simulink model "pendule_simple"  (R2023a)
settings: Solver=VariableStepAuto  StartTime=0.0  StopTime=10.0  RelTol=1e-3
undefined symbols (not defined in the file): g, l
settings Model: Creator=crt4254  LastModifiedBy=crt4254

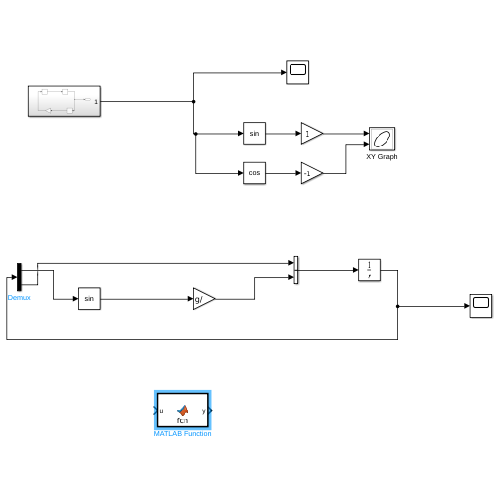
[thumbnail: Simulink's stored preview of the top-level diagram]
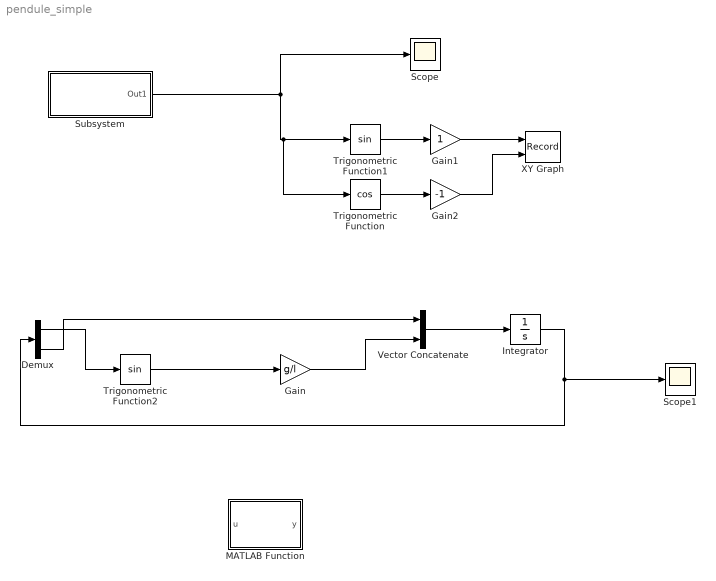
== system pendule_simple ==
  Demux : Demux  Outputs=2
  Gain : Gain  Gain=g/l
  Gain1 : Gain
  Gain2 : Gain  Gain=-1
  Integrator : Integrator  InitialCondition=[1 pi]
  MATLAB Function : MATLAB Function  TreatAsAtomicUnit=on
  Scope : Scope
  Scope1 : Scope
  Subsystem : Subsystem
  Trigonometric Function : Trigonometry  Operator=cos
  Trigonometric Function1 : Trigonometry
  Trigonometric Function2 : Trigonometry
  Vector Concatenate : Concatenate
  XY Graph : Record  FileSettingsInternal="{\"entries\":[{\"content\":{\"excelSettings\":{\"content\":{},\"type\":\"Streamout.ExcelSettings\"}},\"type\":\"Streamout.FileSettingStorage\",\"uuid\":\"855e007d-fd6a-4001-b943-7c5d9cd4a3f9\"}],\"packageUris\":[\"http://schema.mathworks.com/mf0/streamout_blocks/R2020a\"],\"version\":\"1.0\"}"  Layout=[1 1]  SignalsInternal="{\"entries\":[{\"content\":{\"signals\":[{\"content\":{\"blockPath\":[\"pendule_simple/XY Graph\"],\"dimensions\":[1],\"domain\":\"pendule_simple/XY Graph\",\"lineColor\":\"#a2142f\",\"plots\":[1],\"port\":1,\"sid\":[\"\"],\"signalID\":149,\"signalName\":\"Gain1\"},\"type\":\"RecordBlkView.Signal\",\"uuid\":\"53e22b2f-952e-4340-82ff-a1eee0395188\"},{\"content\":{\"blockPath\":[\"pendule_simple/XY Graph\"],\"dimensions\":[1],\"domain\":\"pendule_simple/XY Graph\",\"lineColor\":\"#139fff\",\"plots\":[1],\"port\":2,\"sid\":[\"\"],\"signalID\":153,\"signalName\":\"Gain2\"},\"type\":\"RecordBlkView.Signal\",\"uuid\":\"6553753f-2e0c-4b72-809f-a3ac0624885e\"}]},\"type\":\"RecordBlkView.InputSignals\",\"uuid\":\"8b61cead-f2ec-4eec-bad4-7556f19c9db5\"}],\"packageUris\":[\"http://schema.mathworks.com/mf0/streamout_blocks/R2020a\"],\"version\":\"1.0\"}"  VisualizationBindings="{\"xyplotplugin\":{\"info\":[{\"series\":[{\"bindingParametersList\":[{\"parameter\":\"X-Axis\",\"signalID\":149,\"signalName\":\"Gain1\"},{\"parameter\":\"Y-Axis\",\"signalID\":153,\"signalName\":\"Gain2\"}],\"seriesID\":41298}],\"subplotID\":1}]}}"  CompatibilityTag=XY
  wires:
  Trigonometric Function/1 -> Gain2/1
  Trigonometric Function1/1 -> Gain1/1
  Gain1/1 -> XY Graph/1
  Gain2/1 -> XY Graph/2
  Subsystem/1(Out1) -> Trigonometric Function/1, Trigonometric Function1/1, Scope/1
  Demux/2 -> Vector Concatenate/1
  Demux/1 -> Trigonometric Function2/1
  Trigonometric Function2/1 -> Gain/1
  Gain/1 -> Vector Concatenate/2
  Vector Concatenate/1 -> Integrator/1
  Integrator/1 -> Scope1/1, Demux/1

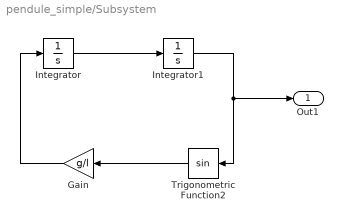
== system pendule_simple/Subsystem ==
  Gain : Gain  Gain=g/l
  Integrator : Integrator  InitialCondition=1
  Integrator1 : Integrator  InitialCondition=pi
  Trigonometric Function2 : Trigonometry
  Out1 : Outport
  wires:
  Integrator1/1 -> Out1/1, Trigonometric Function2/1
  Gain/1 -> Integrator/1
  Trigonometric Function2/1 -> Gain/1
  Integrator/1 -> Integrator1/1

== matlab function pendule_simple/MATLAB Function ==
  data: u input; y output
function y = fcn(u)

y = u;
